simulink model "tracking2024"  (R2023b)
settings: Solver=FixedStepDiscrete  StartTime=0.0  StopTime=inf  FixedStep=0.01  RelTol=1e-3  EnableMultiTasking=on
undefined symbols (not defined in the file): Angular, Linear
libraries: robotlib x6
settings Model: Creator=The MathWorks, Inc.  LastModifiedBy=balaji
settings SolverCC: AlgebraicLoopSolver=TrustRegion
settings DataIOCC: LimitDataPoints=on  SaveFormat=Array  ReturnWorkspaceOutputs=off
settings OptimizationCC: ZeroExternalMemoryAtStartup=off  ZeroInternalMemoryAtStartup=off  LifeSpan=1  MaxStackSize=64
settings DebuggingCC: SolverPrmCheckMsg=warning  UnconnectedInputMsg=warning  UnconnectedOutputMsg=warning  UnconnectedLineMsg=warning  SFUnexpectedBacktrackingDiag=warning  SFNoUnconditionalDefaultTransitionDiag=warning  SFExecutionAtInitializationDiag=none  ArithmeticOperatorsInVariantConditions=warning
settings HardwareCC: ProdBitPerPointer=32  ProdBitPerSizeT=32  ProdBitPerPtrDiffT=32  ProdLargestAtomicFloat=None  ProdIntDivRoundTo=Undefined  ProdEndianess=Unspecified  ProdWordSize=32  ProdHWDeviceType=Generic->Unspecified (assume 32-bit Generic)  TargetHWDeviceType=Generic->Unspecified (assume 32-bit Generic)  UseEmbeddedCoderFeatures=off
settings ModelReferenceCC: EnableRefExpFcnMdlSchedulingChecks=on  PropagateSignalLabelsOutOfModel=off
settings SFSimCC: SimUseLocalCustomCode=off  CustomCodeUndefinedFunction=UseInterfaceOnly  SimTargetLang=C++
settings RTWCC: Description=Embedded Coder  SystemTargetFile=ert.tlc  HardwareBoard=Robot Operating System (ROS)  TLCOptions=-aInlineSetEventsForThisBaseRateFcn=TLC_FALSE -aSuppressMultiTaskScheduler=TLC_FALSE -aRateBasedStepFcn=0  TemplateMakefile=ert_default_tmf  RTWUseLocalCustomCode=off  Toolchain=Catkin  TargetLang=C++
settings CodeAppCC: StateflowObjectComments=on
settings ERTTargetCC: MultiwordLength=2048  ERTCustomFileBanners=off  CodeInterfacePackaging=C++ class  SupportContinuousTime=on  SupportNonInlinedSFcns=on  RemoveResetFunc=off  SupportVariableSizeSignals=on  ModelStepFunctionPrototypeControlCompliant=off  RootIOFormat=Structure reference  ConvertIfToSwitch=off  SuppressUnreachableDefaultCases=off
settings ConfigComp: CovMetricSettings=dw  CovSaveCumulativeToWorkspaceVar=on  CovSaveSingleToWorkspaceVar=on  CovExternalEMLEnable=off  CovSFcnEnable=off

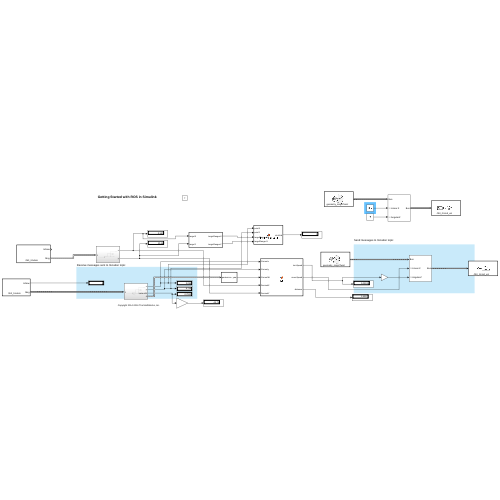
[thumbnail: Simulink's stored preview of the top-level diagram]
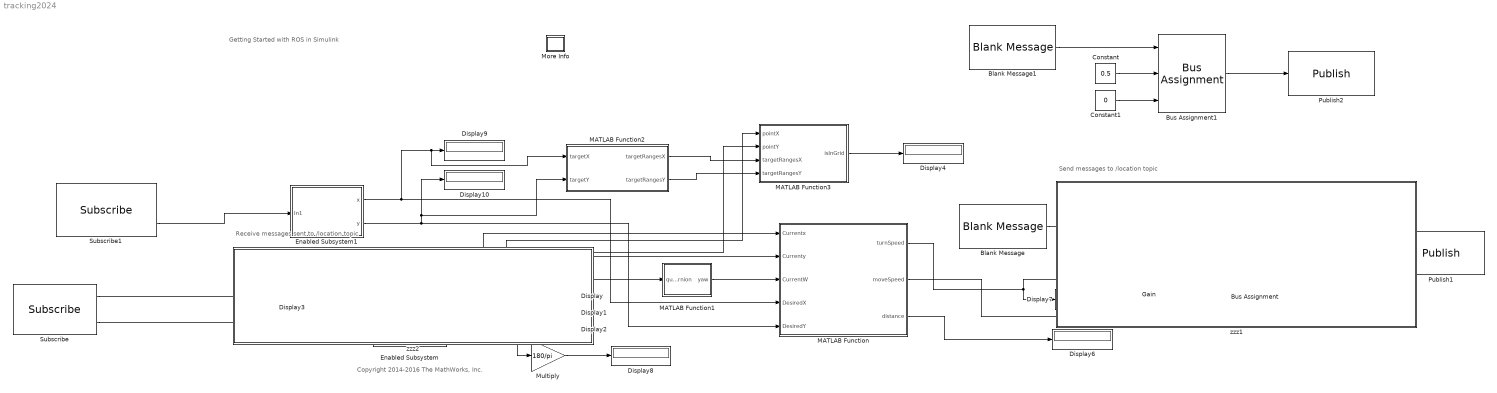
== system tracking2024 ==
  note: Receive messages sent to /location topic
  note: Getting Started with ROS in Simulink
  note: Copyright 2014-2016 The MathWorks, Inc.
  note: Send messages to /location topic
  Blank Message : robotlib/Blank Message  messageClass=Message  entityType=geometry_msgs/Twist  messageType=geometry_msgs/Twist  SampleTime=-1  legacyBusStruct=off
  Blank Message1 : robotlib/Blank Message  messageClass=Message  entityType=geometry_msgs/Twist  messageType=geometry_msgs/Twist  SampleTime=-1  legacyBusStruct=off
  Bus Assignment : BusAssignment  AssignedSignals=Linear.X,Angular.Z
  Bus Assignment1 : BusAssignment  AssignedSignals=Linear.X,Angular.Z
  Constant : Constant  Value=0.5  SampleTime=-1
  Constant1 : Constant  Value=0
  Display{,1..4,6..10} (10 alike) : Display
  Enabled Subsystem : Subsystem
  Enabled Subsystem1 : Subsystem
  Gain : Gain
  MATLAB Function : MATLAB Function  TreatAsAtomicUnit=on
  MATLAB Function1 : MATLAB Function  TreatAsAtomicUnit=on
  MATLAB Function2 : MATLAB Function  TreatAsAtomicUnit=on
  MATLAB Function3 : MATLAB Function  TreatAsAtomicUnit=on
  More Info : Subsystem
      settings: OpenFcn=showdemo(bdroot(gcb))
      mask Display: disp('?')
  Multiply : Gain  Gain=180/pi
  Publish1 : robotlib/Publish  topicSource=Select from ROS network  topic=/tb3_1/cmd_vel  messageType=geometry_msgs/Twist  legacyBusStruct=off  messageQueueLength=105
  Publish2 : robotlib/Publish  topicSource=Select from ROS network  topic=/tb3_0/cmd_vel  messageType=geometry_msgs/Twist  legacyBusStruct=off  messageQueueLength=105
  Subscribe : robotlib/Subscribe  topicSource=Select from ROS network  topic=/tb3_1/odom  messageType=nav_msgs/Odometry  SampleTime=-1  legacyBusStruct=off  messageQueueLength=1
  Subscribe1 : robotlib/Subscribe  topicSource=Select from ROS network  topic=/tb3_0/odom  messageType=nav_msgs/Odometry  SampleTime=-1  legacyBusStruct=off  messageQueueLength=1
  zzz1 : Subsystem  TreatAsAtomicUnit=on
      settings: OpenFcn=% no-op
      mask Display: disp('')
  zzz2 : Subsystem  TreatAsAtomicUnit=on
      settings: OpenFcn=% no-op
      mask Display: disp('')
  wires:
  Bus Assignment/1 -> Publish1/1
  Subscribe/2 -> Enabled Subsystem/1(In1)
  Enabled Subsystem/1(x) -> MATLAB Function/1(Currentx), MATLAB Function3/1(pointX), Display/1
  Enabled Subsystem/2(y) -> MATLAB Function/2(Currenty), MATLAB Function3/2(pointY), Display1/1
  Blank Message/1 -> Bus Assignment/1
  Subscribe/1 -> Display3/1
  MATLAB Function/1(turnSpeed) -> Display7/1, Gain/1
  Multiply/1 -> Display8/1
  Gain/1 -> Bus Assignment/3
  Enabled Subsystem/3(currentW) -> Multiply/1, Display2/1
  MATLAB Function1/1(yaw) -> MATLAB Function/3(CurrentW)
  Enabled Subsystem/4(Output) -> MATLAB Function1/1(quaternion)
  MATLAB Function/2(moveSpeed) -> Bus Assignment/2
  MATLAB Function/3(distance) -> Display6/1
  Subscribe1/2 -> Enabled Subsystem1/1(In1)
  Enabled Subsystem1/1(x) -> MATLAB Function2/1(targetX), Display9/1, MATLAB Function/4(DesiredX)
  Enabled Subsystem1/2(y) -> MATLAB Function2/2(targetY), Display10/1, MATLAB Function/5(DesiredY)
  Bus Assignment1/1 -> Publish2/1
  Blank Message1/1 -> Bus Assignment1/1
  Constant/1 -> Bus Assignment1/2
  Constant1/1 -> Bus Assignment1/3
  MATLAB Function3/1(isInGrid) -> Display4/1
  MATLAB Function2/2(targetRangesY) -> MATLAB Function3/4(targetRangesY)
  MATLAB Function2/1(targetRangesX) -> MATLAB Function3/3(targetRangesX)

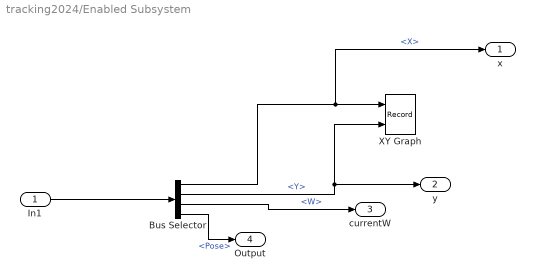
== system tracking2024/Enabled Subsystem ==
  In1 : Inport
  Bus Selector : BusSelector  OutputSignals=Pose.Pose.Position.X,Pose.Pose.Position.Y,Pose.Pose.Orientation.W,Pose.Pose
  XY Graph : Record  FileSettingsInternal="{\"entries\":[{\"content\":{\"excelSettings\":{\"content\":{},\"type\":\"Streamout.ExcelSettings\"}},\"type\":\"Streamout.FileSettingStorage\",\"uuid\":\"\"}],\"packageUris\":[\"http:\\/\\/schema.mathworks.com\\/mf0\\/streamout_blocks\\/R2020a\"],\"version\":\"1.0\"}"  Layout=[1 1]  SignalsInternal="{\"entries\":[{\"content\":{\"signals\":[{\"content\":{\"blockPath\":[],\"dimensions\":[1],\"domain\":\"\",\"lineColor\":\"#4dbeee\",\"plots\":[1],\"port\":1,\"signalID\":16,\"signalName\":\"<X>\"},\"type\":\"RecordBlkView.Signal\",\"uuid\":\"\"},{\"content\":{\"blockPath\":[],\"dimensions\":[1],\"domain\":\"\",\"lineColor\":\"#139fff\",\"plots\":[1],\"port\":2,\"signalID\":19,\"signalName\":\"<Y>\"},\"type\":\"RecordBlkView.Signal\",\"uuid\":\"\"}]},\"type\":\"RecordBlkView.InputSignals\",\"uuid\":\"\"}],\"packageUris\":[\"http:\\/\\/schema.mathworks.com\\/mf0\\/streamout_blocks\\/R2020a\"],\"version\":\"1.0\"}"  VisualizationBindings="{\"xyplotplugin\":{\"info\":[{\"series\":[{\"bindingParametersList\":[{\"parameter\":\"X-Axis\",\"signalID\":16,\"signalName\":\"<X>\"},{\"parameter\":\"Y-Axis\",\"signalID\":19,\"signalName\":\"<Y>\"}],\"seriesID\":27971}],\"subplotID\":1}]}}"  CompatibilityTag=XY  st=-1
  x : Outport  VectorParamsAs1DForOutWhenUnconnected=off
  y : Outport  Port=2  VectorParamsAs1DForOutWhenUnconnected=off
  currentW : Outport  Port=3  VectorParamsAs1DForOutWhenUnconnected=off
  Output : Outport  Port=4
  wires:
  Bus Selector/1 -> x/1, XY Graph/1  "<X>"
  Bus Selector/2 -> XY Graph/2, y/1  "<Y>"
  Bus Selector/3 -> currentW/1  "<W>"
  In1/1 -> Bus Selector/1
  Bus Selector/4 -> Output/1  "<Pose>"

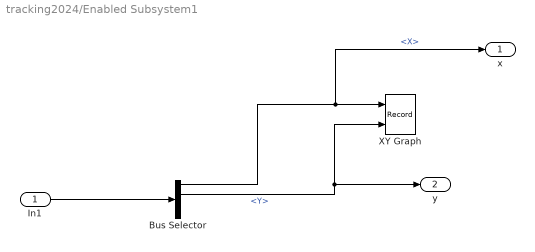
== system tracking2024/Enabled Subsystem1 ==
  In1 : Inport
  Bus Selector : BusSelector  OutputSignals=Pose.Pose.Position.X,Pose.Pose.Position.Y,Pose.Pose.Orientation.W,Pose.Pose
  XY Graph : Record  FileSettingsInternal="{\"entries\":[{\"content\":{\"excelSettings\":{\"content\":{},\"type\":\"Streamout.ExcelSettings\"}},\"type\":\"Streamout.FileSettingStorage\",\"uuid\":\"\"}],\"packageUris\":[\"http:\\/\\/schema.mathworks.com\\/mf0\\/streamout_blocks\\/R2020a\"],\"version\":\"1.0\"}"  Layout=[1 1]  SignalsInternal="{\"entries\":[{\"content\":{\"signals\":[{\"content\":{\"blockPath\":[],\"dimensions\":[1],\"domain\":\"\",\"lineColor\":\"#4dbeee\",\"plots\":[1],\"port\":1,\"signalID\":8,\"signalName\":\"<X>\"},\"type\":\"RecordBlkView.Signal\",\"uuid\":\"\"},{\"content\":{\"blockPath\":[],\"dimensions\":[1],\"domain\":\"\",\"lineColor\":\"#139fff\",\"plots\":[1],\"port\":2,\"signalID\":11,\"signalName\":\"<Y>\"},\"type\":\"RecordBlkView.Signal\",\"uuid\":\"\"}]},\"type\":\"RecordBlkView.InputSignals\",\"uuid\":\"\"}],\"packageUris\":[\"http:\\/\\/schema.mathworks.com\\/mf0\\/streamout_blocks\\/R2020a\"],\"version\":\"1.0\"}"  VisualizationBindings="{\"xyplotplugin\":{\"info\":[{\"series\":[{\"bindingParametersList\":[{\"parameter\":\"X-Axis\",\"signalID\":8,\"signalName\":\"<X>\"},{\"parameter\":\"Y-Axis\",\"signalID\":11,\"signalName\":\"<Y>\"}],\"seriesID\":32689}],\"subplotID\":1}]}}"  CompatibilityTag=XY  st=-1
  x : Outport  VectorParamsAs1DForOutWhenUnconnected=off
  y : Outport  Port=2  VectorParamsAs1DForOutWhenUnconnected=off
  wires:
  Bus Selector/1 -> x/1, XY Graph/1  "<X>"
  Bus Selector/2 -> XY Graph/2, y/1  "<Y>"
  In1/1 -> Bus Selector/1

== system tracking2024/More Info ==

== system tracking2024/zzz1 ==

== system tracking2024/zzz2 ==

== matlab function tracking2024/MATLAB Function1 ==
  data: quaternion input; yaw output
function yaw = getYawFromQuaternion(quaternion)
    % Check if quaternion is valid
    if ~isfield(quaternion, 'Orientation')
        error('Invalid quaternion structure. Make sure it has the ''Orientation'' field.');
    end

    % Extract quaternion components
    quat = [quaternion.Orientation.X, quaternion.Orientation.Y, quaternion.Orientation.Z, quaternion.Orientation.W];

    % Use quat2eul to convert quaternion to Euler angles (roll, pitch, yaw)
    euler_angles = quat2eul(quat);

    % Extract the yaw angle (third element of the Euler angles)
    yaw = euler_angles(3);
end

== matlab function tracking2024/MATLAB Function ==
  data: Currentx input; turnSpeed output; Currenty input; CurrentW input; DesiredX input; DesiredY input; moveSpeed output; distance output
function [turnSpeed, moveSpeed,distance] = fcn(Currentx, Currenty, CurrentW, DesiredX, DesiredY)

    targetAngle = atan2(DesiredY - Currenty, DesiredX - Currentx);

    distance = sqrt((DesiredX - Currentx)^2 + (DesiredY - Currenty)^2);

    angleDifference = targetAngle - CurrentW;

    angleDifference = mod(angleDifference + pi, 2*pi) - pi;

    if abs(angleDifference) < 0.03
        turnSpeed = 0;
        if distance <  0.1
            moveSpeed = 0;
        else
            moveSpeed = min(0.5, distance);
        end
    else
        
        turnSpeed = angleDifference;
        
        moveSpeed = min(0.5, distance) * 1.25;
    end
end

== matlab function tracking2024/MATLAB Function2 ==
  data: targetX input; targetRangesX output; targetY input; targetRangesY output
function [targetRangesX, targetRangesY]  = fcn(targetX, targetY)

x_center = targetX;
y_center = targetY;

radius = 1;

theta = linspace(0, 2*pi, 100);

targetRangesX = x_center + radius * cos(theta);
targetRangesY = y_center + radius * sin(theta);

    plot(targetRangesX, targetRangesY, 'b');
    hold on; 

    axis equal;
    xlabel('X Coordinates');
    ylabel('Y Coordinates');
    title('Current Boundary Region Created by the Target Robot');
    grid on;
end

== matlab function tracking2024/MATLAB Function3 ==
  data: pointX input; isInGrid output; pointY input; targetRangesX input; targetRangesY input
function isInGrid = checkPointInGrid(pointX, pointY, targetRangesX, targetRangesY)
    minX = min(targetRangesX(:));
    maxX = max(targetRangesX(:));
    minY = min(targetRangesY(:));
    maxY = max(targetRangesY(:));

    isInGrid = (pointX >= minX && pointX <= maxX) && (pointY >= minY && pointY <= maxY);
end
